simulink library "device_library"  (R2021b)
settings: Solver=VariableStepAuto  StartTime=0.0  StopTime=10.0  RelTol=1e-3
undefined symbols (not defined in the file or in its folder): base
libraries: spsControlledVoltageSourceLib x15, spsThreePhaseVIMeasurementLib x10, spsabctodq0Lib x10, $bdroot x6, spsThreePhaseSeriesRLCBranchLib x5, spsdq0toabcLib x3
settings Model: Creator=lpwoolcock  LastModifiedBy=lukew
settings SolverCC: AlgebraicLoopSolver=TrustRegion
settings DebuggingCC: SFMachineParentedDataDiag=warning

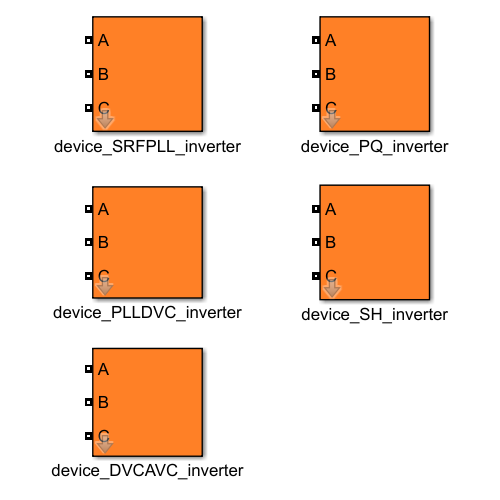
[thumbnail: Simulink's stored preview of the top-level diagram]
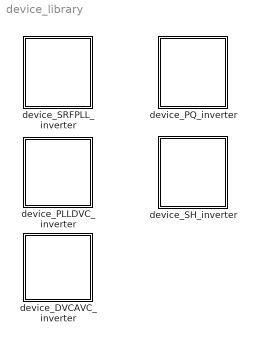
== system device_library ==
  device_DVCAVC_inverter : Subsystem  mask{Rf=0, Lf=0, Cdc=0, K_p_acc=0, K_i_acc=0, K_p_pll=0, K_i_pll=0, K_p_dvc=0, K_i_dvc=0, K_p_avc=0, K_i_avc=0, Psrc=0, Vref=0, K_droop=0}
      mask Display: patch([0 1 1 0], [0 0 1 1], [1 0.5 0.15])
  device_PLLDVC_inverter : Subsystem  mask{Rf=0, Lf=0, K_p_pll=0, K_i_pll=0, K_p_acc=0, K_i_acc=0, K_p_dvc=0, K_i_dvc=0, Psrc=0, Iq=0, Cdc=0}
      mask Display: patch([0 1 1 0], [0 0 1 1], [1 0.5 0.15])
  device_PQ_inverter : Subsystem  mask{Rf=0, Lf=0, S0=0, phi=0, K_p_pll=0, K_i_pll=0, K_p_acc=0, K_i_acc=0, K_p_P=0, K_i_P=0}
      mask Display: patch([0 1 1 0], [0 0 1 1], [1 0.5 0.15])
  device_SH_inverter : Subsystem  mask{Rf=0, Lf=0, P0=0, Q0=0, tau_rms=0, K_p_pll=0, K_i_pll=0, K_p_acc=0, K_i_acc=0}
      mask Display: patch([0 1 1 0], [0 0 1 1], [1 0.5 0.15])
  device_SRFPLL_inverter : Subsystem  mask{Rf=0, Lf=0, Iref=0, phi=0, K_p_pll=0, K_i_pll=0, K_p_acc=0, K_i_acc=0}
      mask prompts: Iref "I0"
      mask Display: patch([0 1 1 0], [0 0 1 1], [1 0.5 0.15])

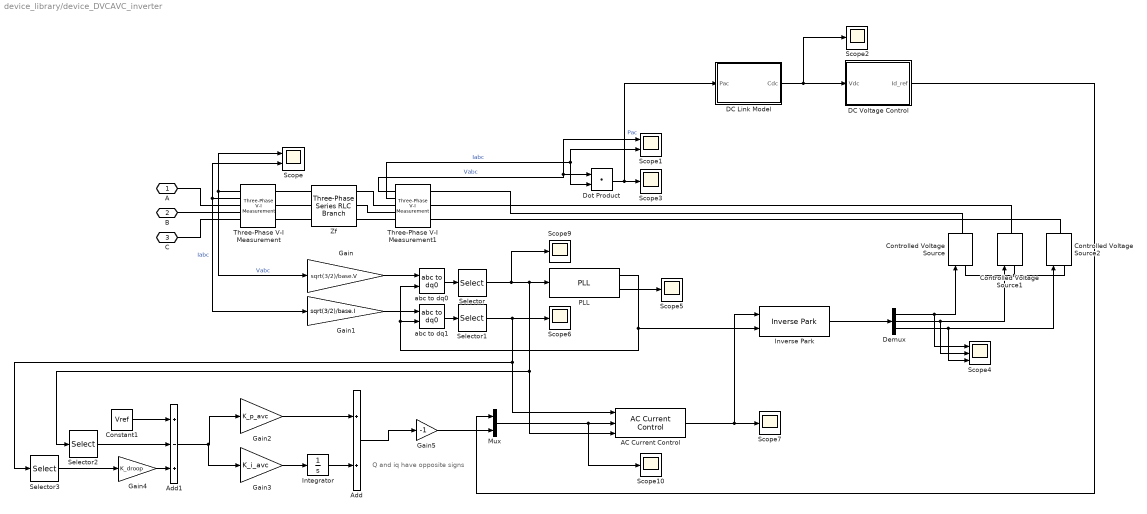
== system device_library/device_DVCAVC_inverter ==
  note: Q and iq have opposite signs
  AC Current Control : $bdroot/device_SRFPLL_inverter/AC Current Control  SystemSampleTime=-1  VariantActivationTime=update diagram  Latency=0  AutoFrameSizeCalculation=off
  Add : Sum
  Add1 : Sum  Inputs=+-+
  Constant1 : Constant  Value=Vref
  Controlled Voltage Source : spsControlledVoltageSourceLib/Controlled Voltage Source  Initialize=on  Source_Type=AC  Amplitude=0  Phase=0  Frequency=0  Measurements=None
  Controlled Voltage Source1 : spsControlledVoltageSourceLib/Controlled Voltage Source  Initialize=on  Source_Type=AC  Amplitude=0  Phase=0  Frequency=0  Measurements=None
  Controlled Voltage Source2 : spsControlledVoltageSourceLib/Controlled Voltage Source  Initialize=on  Source_Type=AC  Amplitude=0  Phase=0  Frequency=0  Measurements=None
  DC Link Model : Subsystem
  DC Voltage Control : Subsystem
  Demux : Demux  Outputs=3
  Dot Product : DotProduct  InputSameDT=on  OutDataTypeStr=Inherit: Inherit via internal rule
  Gain : Gain  Gain=sqrt(3/2)/base.V
  Gain1 : Gain  Gain=sqrt(3/2)/base.I
  Gain2 : Gain  Gain=K_p_avc
  Gain3 : Gain  Gain=K_i_avc
  Gain4 : Gain  Gain=K_droop
  Gain5 : Gain  Gain=-1
  Integrator : Integrator
  Inverse Park : $bdroot/device_SRFPLL_inverter/Inverse Park  SystemSampleTime=-1  VariantActivationTime=update diagram  Latency=0  AutoFrameSizeCalculation=off
  Mux : Mux  Inputs=2
  PLL : $bdroot/device_SRFPLL_inverter/PLL  SystemSampleTime=-1  VariantActivationTime=update diagram  Latency=0  AutoFrameSizeCalculation=off
  Scope : Scope  NumInputPorts=2
  Scope1 : Scope  NumInputPorts=2
  Scope{2..3,5..7,9..10} (7 alike) : Scope
  Scope4 : Scope  NumInputPorts=3
  Selector : Selector  InputPortWidth=3  IndexOptions=Index vector (dialog)  Indices=[1 2]  OutputSizes=1
  Selector1 : Selector  InputPortWidth=3  IndexOptions=Index vector (dialog)  Indices=[1 2]  OutputSizes=1
  Selector2 : Selector  InputPortWidth=2  IndexOptions=Index vector (dialog)  Indices=[1]  OutputSizes=1
  Selector3 : Selector  InputPortWidth=2  IndexOptions=Index vector (dialog)  Indices=[2]  OutputSizes=1
  Three-Phase V-I Measurement : spsThreePhaseVIMeasurementLib/Three-Phase V-I Measurement  VoltageMeasurement=phase-to-ground  SetLabelV=off  LabelV=Vabc  Vpu=off  VpuLL=off  CurrentMeasurement=yes  SetLabelI=off  LabelI=Iabc  Ipu=off  Pbase=100e6  Vbase=500e3  OutputType=Complex  PhasorSimulation=off  PSBequivalent=0
  Three-Phase V-I Measurement1 : spsThreePhaseVIMeasurementLib/Three-Phase V-I Measurement  VoltageMeasurement=phase-to-ground  SetLabelV=off  LabelV=Vabc  Vpu=off  VpuLL=off  CurrentMeasurement=yes  SetLabelI=off  LabelI=Iabc  Ipu=off  Pbase=100e6  Vbase=500e3  OutputType=Complex  PhasorSimulation=off  PSBequivalent=0
  Zf : spsThreePhaseSeriesRLCBranchLib/Three-Phase Series RLC Branch  LConnTagsString=A|B|C  RConnTagsString=A|B|C  BranchType=RL  Resistance=Rf*base.Z  Inductance=Lf*base.L  Capacitance=1e-6  Measurements=None
  abc to dq0 : spsabctodq0Lib/abc to dq0  Alignment=90 degrees behind phase A axis
  abc to dq1 : spsabctodq0Lib/abc to dq0  Alignment=90 degrees behind phase A axis
  "A " : PMIOPort  Side=Left
  B : PMIOPort  Port=2  Side=Left
  C : PMIOPort  Port=3  Side=Left
  wires:
  AC Current Control/1 -> Inverse Park/1, Scope7/1
  Gain1/1 -> abc to dq1/1
  Three-Phase V-I Measurement/1 -> Gain/1, Scope/1  "Vabc"
  DC Voltage Control/1(Id_ref) -> Mux/1
  Add/1 -> Gain5/1
  abc to dq0/1 -> Selector/1
  Gain3/1 -> Integrator/1
  Constant1/1 -> Add1/1
  Dot Product/1 -> Scope3/1, DC Link Model/1(Pac)  "Pac"
  Selector3/1 -> Gain4/1
  Demux/1 -> Controlled Voltage Source/1, Scope4/1
  Selector/1 -> PLL/1, AC Current Control/3, Selector2/1, Scope9/1
  PLL/2 -> Scope5/1
  Three-Phase V-I Measurement/2 -> Gain1/1, Scope/2  "Iabc"
  PLL/1 -> Inverse Park/2, abc to dq0/2, abc to dq1/2
  Demux/3 -> Controlled Voltage Source2/1, Scope4/3
  abc to dq1/1 -> Selector1/1
  Three-Phase V-I Measurement1/2 -> Dot Product/2, Scope1/2  "Iabc"
  Demux/2 -> Controlled Voltage Source1/1, Scope4/2
  Gain5/1 -> Mux/2
  Mux/1 -> AC Current Control/2, Scope10/1
  Three-Phase V-I Measurement1/1 -> Dot Product/1, Scope1/1  "Vabc"
  Gain2/1 -> Add/1
  Gain4/1 -> Add1/3
  Selector2/1 -> Add1/2
  Integrator/1 -> Add/2
  Gain/1 -> abc to dq0/1
  Inverse Park/1 -> Demux/1
  Selector1/1 -> Scope6/1, AC Current Control/1, Selector3/1
  DC Link Model/1(Cdc) -> DC Voltage Control/1(Vdc), Scope2/1
  Add1/1 -> Gain2/1, Gain3/1
  connections:
  Controlled Voltage Source2/LConn1 -- Controlled Voltage Source/LConn1 -- Controlled Voltage Source1/LConn1
  Three-Phase V-I Measurement/LConn3 -- Zf/LConn3
  C/RConn1 -- Three-Phase V-I Measurement/RConn3
  Zf/RConn3 -- Three-Phase V-I Measurement1/RConn3
  Three-Phase V-I Measurement1/LConn2 -- Controlled Voltage Source1/RConn1
  B/RConn1 -- Three-Phase V-I Measurement/RConn2
  Three-Phase V-I Measurement/LConn2 -- Zf/LConn2
  Zf/RConn1 -- Three-Phase V-I Measurement1/RConn1
  Three-Phase V-I Measurement1/LConn3 -- Controlled Voltage Source2/RConn1
  Three-Phase V-I Measurement1/LConn1 -- Controlled Voltage Source/RConn1
  Zf/RConn2 -- Three-Phase V-I Measurement1/RConn2
  "A "/RConn1 -- Three-Phase V-I Measurement/RConn1
  Three-Phase V-I Measurement/LConn1 -- Zf/LConn1

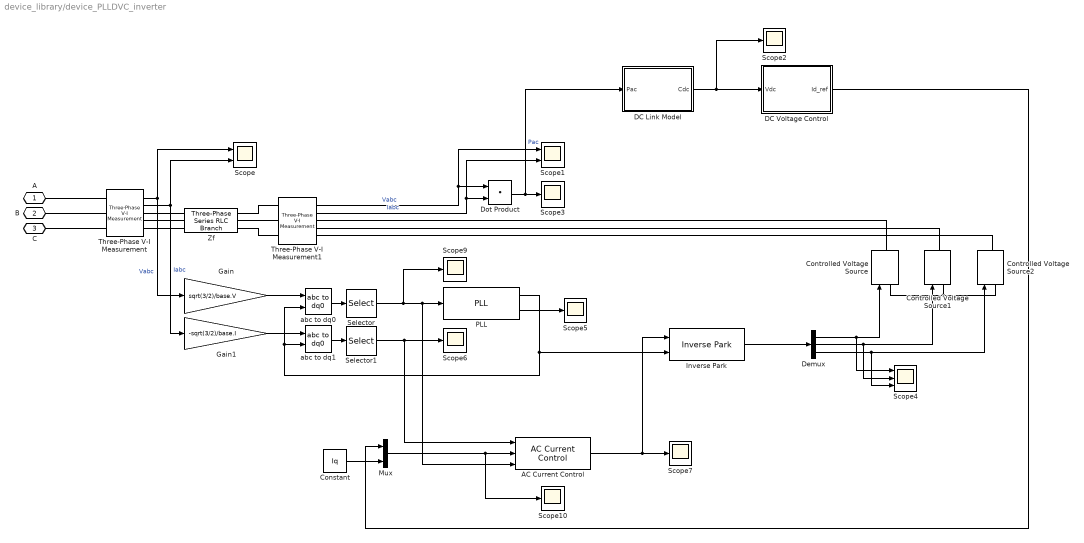
== system device_library/device_PLLDVC_inverter ==
  AC Current Control : $bdroot/device_SRFPLL_inverter/AC Current Control  SystemSampleTime=-1  VariantActivationTime=update diagram  Latency=0  AutoFrameSizeCalculation=off
  Constant : Constant  Value=Iq
  Controlled Voltage Source : spsControlledVoltageSourceLib/Controlled Voltage Source  Initialize=on  Source_Type=AC  Amplitude=0  Phase=0  Frequency=0  Measurements=None
  Controlled Voltage Source1 : spsControlledVoltageSourceLib/Controlled Voltage Source  Initialize=on  Source_Type=AC  Amplitude=0  Phase=0  Frequency=0  Measurements=None
  Controlled Voltage Source2 : spsControlledVoltageSourceLib/Controlled Voltage Source  Initialize=on  Source_Type=AC  Amplitude=0  Phase=0  Frequency=0  Measurements=None
  DC Link Model : Subsystem
  DC Voltage Control : Subsystem
  Demux : Demux  Outputs=3
  Dot Product : DotProduct  InputSameDT=on  OutDataTypeStr=Inherit: Inherit via internal rule
  Gain : Gain  Gain=sqrt(3/2)/base.V
  Gain1 : Gain  Gain=-sqrt(3/2)/base.I
  Inverse Park : $bdroot/device_SRFPLL_inverter/Inverse Park  SystemSampleTime=-1  VariantActivationTime=update diagram  Latency=0  AutoFrameSizeCalculation=off
  Mux : Mux  Inputs=2
  PLL : $bdroot/device_SRFPLL_inverter/PLL  SystemSampleTime=-1  VariantActivationTime=update diagram  Latency=0  AutoFrameSizeCalculation=off
  Scope : Scope  NumInputPorts=2
  Scope1 : Scope  NumInputPorts=2
  Scope{2..3,5..7,9..10} (7 alike) : Scope
  Scope4 : Scope  NumInputPorts=3
  Selector : Selector  InputPortWidth=3  IndexOptions=Index vector (dialog)  Indices=[1 2]  OutputSizes=1
  Selector1 : Selector  InputPortWidth=3  IndexOptions=Index vector (dialog)  Indices=[1 2]  OutputSizes=1
  Three-Phase V-I Measurement : spsThreePhaseVIMeasurementLib/Three-Phase V-I Measurement  VoltageMeasurement=phase-to-ground  SetLabelV=off  LabelV=Vabc  Vpu=off  VpuLL=off  CurrentMeasurement=yes  SetLabelI=off  LabelI=Iabc  Ipu=off  Pbase=100e6  Vbase=500e3  OutputType=Complex  PhasorSimulation=off  PSBequivalent=0
  Three-Phase V-I Measurement1 : spsThreePhaseVIMeasurementLib/Three-Phase V-I Measurement  VoltageMeasurement=phase-to-ground  SetLabelV=off  LabelV=Vabc  Vpu=off  VpuLL=off  CurrentMeasurement=yes  SetLabelI=off  LabelI=Iabc  Ipu=off  Pbase=100e6  Vbase=500e3  OutputType=Complex  PhasorSimulation=off  PSBequivalent=0
  Zf : spsThreePhaseSeriesRLCBranchLib/Three-Phase Series RLC Branch  LConnTagsString=A|B|C  RConnTagsString=A|B|C  BranchType=RL  Resistance=Rf*base.Z  Inductance=Lf*base.L  Capacitance=1e-6  Measurements=None
  abc to dq0 : spsabctodq0Lib/abc to dq0  Alignment=90 degrees behind phase A axis
  abc to dq1 : spsabctodq0Lib/abc to dq0  Alignment=90 degrees behind phase A axis
  "A " : PMIOPort  Side=Left
  B : PMIOPort  Port=2  Side=Left
  C : PMIOPort  Port=3  Side=Left
  wires:
  Constant/1 -> Mux/2
  Selector1/1 -> AC Current Control/1, Scope6/1
  AC Current Control/1 -> Scope7/1, Inverse Park/1
  Mux/1 -> Scope10/1, AC Current Control/2
  Inverse Park/1 -> Demux/1
  Demux/3 -> Scope4/3, Controlled Voltage Source2/1
  Three-Phase V-I Measurement/1 -> Gain/1, Scope/1  "Vabc"
  PLL/1 -> abc to dq1/2, abc to dq0/2, Inverse Park/2
  PLL/2 -> Scope5/1
  Dot Product/1 -> DC Link Model/1(Pac), Scope3/1  "Pac"
  Demux/1 -> Scope4/1, Controlled Voltage Source/1
  Three-Phase V-I Measurement1/1 -> Scope1/1, Dot Product/1  "Vabc"
  DC Link Model/1(Cdc) -> Scope2/1, DC Voltage Control/1(Vdc)
  Three-Phase V-I Measurement/2 -> Scope/2, Gain1/1  "Iabc"
  DC Voltage Control/1(Id_ref) -> Mux/1
  Demux/2 -> Scope4/2, Controlled Voltage Source1/1
  Three-Phase V-I Measurement1/2 -> Dot Product/2, Scope1/2  "Iabc"
  Gain1/1 -> abc to dq1/1
  Gain/1 -> abc to dq0/1
  Selector/1 -> Scope9/1, AC Current Control/3, PLL/1
  abc to dq0/1 -> Selector/1
  abc to dq1/1 -> Selector1/1
  connections:
  Controlled Voltage Source2/LConn1 -- Controlled Voltage Source1/LConn1 -- Controlled Voltage Source/LConn1
  Three-Phase V-I Measurement1/LConn1 -- Zf/RConn1
  B/RConn1 -- Three-Phase V-I Measurement/LConn2
  Three-Phase V-I Measurement/RConn2 -- Zf/LConn2
  Three-Phase V-I Measurement1/RConn2 -- Controlled Voltage Source1/RConn1
  "A "/RConn1 -- Three-Phase V-I Measurement/LConn1
  C/RConn1 -- Three-Phase V-I Measurement/LConn3
  Three-Phase V-I Measurement1/RConn1 -- Controlled Voltage Source/RConn1
  Three-Phase V-I Measurement1/RConn3 -- Controlled Voltage Source2/RConn1
  Zf/RConn3 -- Three-Phase V-I Measurement1/LConn3
  Zf/RConn2 -- Three-Phase V-I Measurement1/LConn2
  Zf/LConn1 -- Three-Phase V-I Measurement/RConn1
  Three-Phase V-I Measurement/RConn3 -- Zf/LConn3

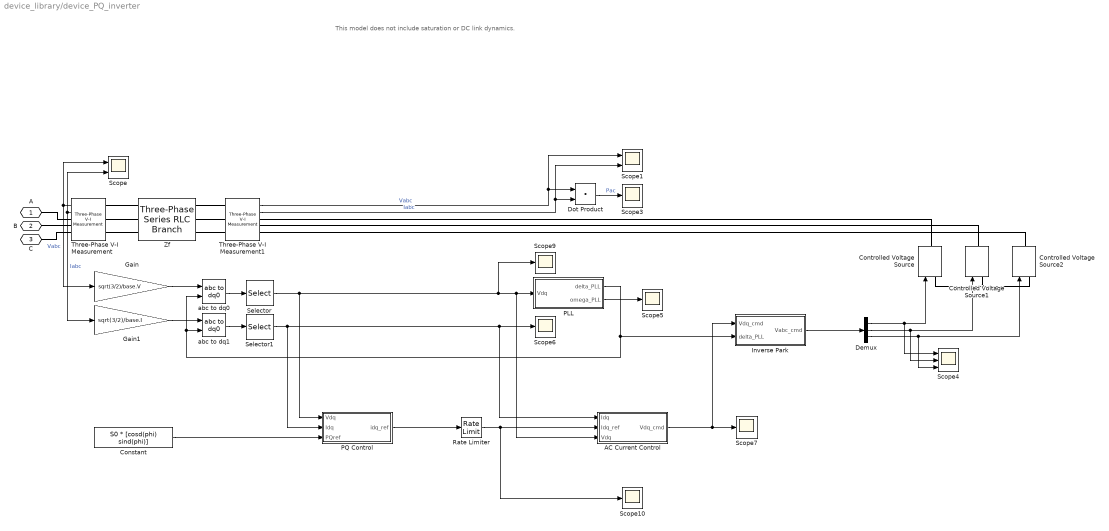
== system device_library/device_PQ_inverter ==
  note: This model does not include saturation or DC link dynamics.
  AC Current Control : Subsystem
  Constant : Constant  Value=S0 * [cosd(phi) sind(phi)]
  Controlled Voltage Source : spsControlledVoltageSourceLib/Controlled Voltage Source  Initialize=on  Source_Type=AC  Amplitude=0  Phase=0  Frequency=0  Measurements=None
  Controlled Voltage Source1 : spsControlledVoltageSourceLib/Controlled Voltage Source  Initialize=on  Source_Type=AC  Amplitude=0  Phase=0  Frequency=0  Measurements=None
  Controlled Voltage Source2 : spsControlledVoltageSourceLib/Controlled Voltage Source  Initialize=on  Source_Type=AC  Amplitude=0  Phase=0  Frequency=0  Measurements=None
  Demux : Demux  Outputs=3
  Dot Product : DotProduct  InputSameDT=on  OutDataTypeStr=Inherit: Inherit via internal rule
  Gain : Gain  Gain=sqrt(3/2)/base.V
  Gain1 : Gain  Gain=sqrt(3/2)/base.I
  Inverse Park : Subsystem
  PLL : Subsystem
  PQ Control : Subsystem
  Rate Limiter : RateLimiter  RisingSlewLimit=1000  FallingSlewLimit=-1000  SampleTimeMode=inherited
  Scope : Scope  NumInputPorts=2
  Scope1 : Scope  NumInputPorts=2
  Scope{3,5..7,9..10} (6 alike) : Scope
  Scope4 : Scope  NumInputPorts=3
  Selector : Selector  InputPortWidth=3  IndexOptions=Index vector (dialog)  Indices=[1 2]  OutputSizes=1
  Selector1 : Selector  InputPortWidth=3  IndexOptions=Index vector (dialog)  Indices=[1 2]  OutputSizes=1
  Three-Phase V-I Measurement : spsThreePhaseVIMeasurementLib/Three-Phase V-I Measurement  VoltageMeasurement=phase-to-ground  SetLabelV=off  LabelV=Vabc  Vpu=off  VpuLL=off  CurrentMeasurement=yes  SetLabelI=off  LabelI=Iabc  Ipu=off  Pbase=100e6  Vbase=500e3  OutputType=Complex  PhasorSimulation=off  PSBequivalent=0
  Three-Phase V-I Measurement1 : spsThreePhaseVIMeasurementLib/Three-Phase V-I Measurement  VoltageMeasurement=phase-to-ground  SetLabelV=off  LabelV=Vabc  Vpu=off  VpuLL=off  CurrentMeasurement=yes  SetLabelI=off  LabelI=Iabc  Ipu=off  Pbase=100e6  Vbase=500e3  OutputType=Complex  PhasorSimulation=off  PSBequivalent=0
  Zf : spsThreePhaseSeriesRLCBranchLib/Three-Phase Series RLC Branch  LConnTagsString=A|B|C  RConnTagsString=A|B|C  BranchType=RL  Resistance=Rf*base.Z  Inductance=Lf*base.L  Capacitance=1e-6  Measurements=None
  abc to dq0 : spsabctodq0Lib/abc to dq0  Alignment=90 degrees behind phase A axis
  abc to dq1 : spsabctodq0Lib/abc to dq0  Alignment=90 degrees behind phase A axis
  A : PMIOPort  Side=Left
  B : PMIOPort  Port=2  Side=Left
  C : PMIOPort  Port=3  Side=Left
  wires:
  Rate Limiter/1 -> AC Current Control/2(Idq_ref), Scope10/1
  Inverse Park/1(Vabc_cmd) -> Demux/1
  abc to dq1/1 -> Selector1/1
  PLL/2(omega_PLL) -> Scope5/1
  abc to dq0/1 -> Selector/1
  Three-Phase V-I Measurement1/1 -> Dot Product/1, Scope1/1  "Vabc"
  Gain/1 -> abc to dq0/1
  Demux/3 -> Controlled Voltage Source2/1, Scope4/3
  Three-Phase V-I Measurement1/2 -> Scope1/2, Dot Product/2  "Iabc"
  AC Current Control/1(Vdq_cmd) -> Inverse Park/1(Vdq_cmd), Scope7/1
  Selector1/1 -> PQ Control/2(Idq), Scope6/1, AC Current Control/1(Idq)
  Dot Product/1 -> Scope3/1  "Pac"
  Demux/1 -> Controlled Voltage Source/1, Scope4/1
  Three-Phase V-I Measurement/1 -> Scope/1, Gain/1  "Vabc"
  Demux/2 -> Controlled Voltage Source1/1, Scope4/2
  Gain1/1 -> abc to dq1/1
  Three-Phase V-I Measurement/2 -> Scope/2, Gain1/1  "Iabc"
  PLL/1(delta_PLL) -> Inverse Park/2(delta_PLL), abc to dq0/2, abc to dq1/2
  Selector/1 -> PQ Control/1(Vdq), PLL/1(Vdq), AC Current Control/3(Vdq), Scope9/1
  Constant/1 -> PQ Control/3(PQref)
  PQ Control/1(idq_ref) -> Rate Limiter/1
  connections:
  Three-Phase V-I Measurement1/LConn1 -- Zf/RConn1
  Three-Phase V-I Measurement1/RConn2 -- Controlled Voltage Source1/RConn1
  Controlled Voltage Source2/LConn1 -- Controlled Voltage Source1/LConn1 -- Controlled Voltage Source/LConn1
  Three-Phase V-I Measurement1/RConn3 -- Controlled Voltage Source2/RConn1
  Zf/RConn3 -- Three-Phase V-I Measurement1/LConn3
  Zf/RConn2 -- Three-Phase V-I Measurement1/LConn2
  Three-Phase V-I Measurement1/RConn1 -- Controlled Voltage Source/RConn1
  A/RConn1 -- Three-Phase V-I Measurement/RConn1
  B/RConn1 -- Three-Phase V-I Measurement/RConn2
  C/RConn1 -- Three-Phase V-I Measurement/RConn3
  Three-Phase V-I Measurement/LConn1 -- Zf/LConn1
  Three-Phase V-I Measurement/LConn2 -- Zf/LConn2
  Three-Phase V-I Measurement/LConn3 -- Zf/LConn3

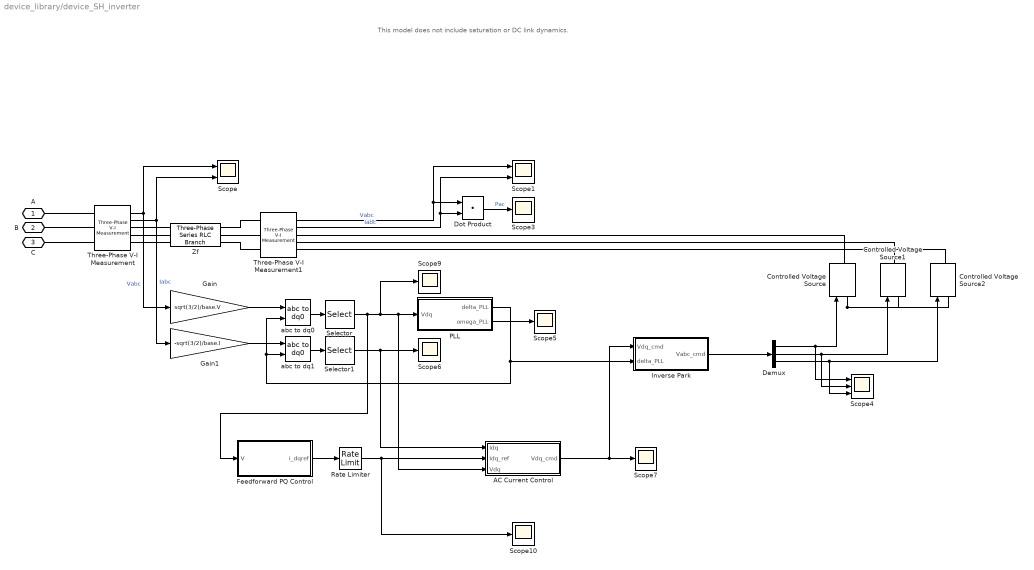
== system device_library/device_SH_inverter ==
  note: This model does not include saturation or DC link dynamics.
  AC Current Control : Subsystem
  Controlled Voltage Source : spsControlledVoltageSourceLib/Controlled Voltage Source  Initialize=on  Source_Type=AC  Amplitude=0  Phase=0  Frequency=0  Measurements=None
  Controlled Voltage Source1 : spsControlledVoltageSourceLib/Controlled Voltage Source  Initialize=on  Source_Type=AC  Amplitude=0  Phase=0  Frequency=0  Measurements=None
  Controlled Voltage Source2 : spsControlledVoltageSourceLib/Controlled Voltage Source  Initialize=on  Source_Type=AC  Amplitude=0  Phase=0  Frequency=0  Measurements=None
  Demux : Demux  Outputs=3
  Dot Product : DotProduct  InputSameDT=on  OutDataTypeStr=Inherit: Inherit via internal rule
  Feedforward PQ Control : Subsystem
  Gain : Gain  Gain=sqrt(3/2)/base.V
  Gain1 : Gain  Gain=-sqrt(3/2)/base.I
  Inverse Park : Subsystem
  PLL : Subsystem
  Rate Limiter : RateLimiter  RisingSlewLimit=1000  FallingSlewLimit=-1000  SampleTimeMode=inherited
  Scope : Scope  NumInputPorts=2
  Scope1 : Scope  NumInputPorts=2
  Scope{3,5..7,9..10} (6 alike) : Scope
  Scope4 : Scope  NumInputPorts=3
  Selector : Selector  InputPortWidth=3  IndexOptions=Index vector (dialog)  Indices=[1 2]  OutputSizes=1
  Selector1 : Selector  InputPortWidth=3  IndexOptions=Index vector (dialog)  Indices=[1 2]  OutputSizes=1
  Three-Phase V-I Measurement : spsThreePhaseVIMeasurementLib/Three-Phase V-I Measurement  VoltageMeasurement=phase-to-ground  SetLabelV=off  LabelV=Vabc  Vpu=off  VpuLL=off  CurrentMeasurement=yes  SetLabelI=off  LabelI=Iabc  Ipu=off  Pbase=100e6  Vbase=500e3  OutputType=Complex  PhasorSimulation=off  PSBequivalent=0
  Three-Phase V-I Measurement1 : spsThreePhaseVIMeasurementLib/Three-Phase V-I Measurement  VoltageMeasurement=phase-to-ground  SetLabelV=off  LabelV=Vabc  Vpu=off  VpuLL=off  CurrentMeasurement=yes  SetLabelI=off  LabelI=Iabc  Ipu=off  Pbase=100e6  Vbase=500e3  OutputType=Complex  PhasorSimulation=off  PSBequivalent=0
  Zf : spsThreePhaseSeriesRLCBranchLib/Three-Phase Series RLC Branch  LConnTagsString=A|B|C  RConnTagsString=A|B|C  BranchType=RL  Resistance=Rf*base.Z  Inductance=Lf*base.L  Capacitance=1e-6  Measurements=None
  abc to dq0 : spsabctodq0Lib/abc to dq0  Alignment=90 degrees behind phase A axis
  abc to dq1 : spsabctodq0Lib/abc to dq0  Alignment=90 degrees behind phase A axis
  A : PMIOPort  Side=Left
  B : PMIOPort  Port=2  Side=Left
  C : PMIOPort  Port=3  Side=Left
  wires:
  Selector/1 -> Feedforward PQ Control/1(V), Scope9/1, AC Current Control/3(Vdq), PLL/1(Vdq)
  PLL/1(delta_PLL) -> abc to dq1/2, abc to dq0/2, Inverse Park/2(delta_PLL)
  Three-Phase V-I Measurement/2 -> Scope/2, Gain1/1  "Iabc"
  Gain1/1 -> abc to dq1/1
  Demux/2 -> Scope4/2, Controlled Voltage Source1/1
  Three-Phase V-I Measurement/1 -> Gain/1, Scope/1  "Vabc"
  Demux/1 -> Scope4/1, Controlled Voltage Source/1
  Dot Product/1 -> Scope3/1  "Pac"
  Selector1/1 -> AC Current Control/1(Idq), Scope6/1
  AC Current Control/1(Vdq_cmd) -> Scope7/1, Inverse Park/1(Vdq_cmd)
  Three-Phase V-I Measurement1/2 -> Dot Product/2, Scope1/2  "Iabc"
  Demux/3 -> Scope4/3, Controlled Voltage Source2/1
  Gain/1 -> abc to dq0/1
  Three-Phase V-I Measurement1/1 -> Scope1/1, Dot Product/1  "Vabc"
  abc to dq0/1 -> Selector/1
  PLL/2(omega_PLL) -> Scope5/1
  abc to dq1/1 -> Selector1/1
  Inverse Park/1(Vabc_cmd) -> Demux/1
  Rate Limiter/1 -> Scope10/1, AC Current Control/2(Idq_ref)
  Feedforward PQ Control/1(i_dqref) -> Rate Limiter/1
  connections:
  Three-Phase V-I Measurement1/RConn1 -- Controlled Voltage Source/RConn1
  A/RConn1 -- Three-Phase V-I Measurement/LConn1
  Zf/RConn2 -- Three-Phase V-I Measurement1/LConn2
  Three-Phase V-I Measurement/RConn2 -- Zf/LConn2
  B/RConn1 -- Three-Phase V-I Measurement/LConn2
  Zf/RConn3 -- Three-Phase V-I Measurement1/LConn3
  Three-Phase V-I Measurement1/RConn3 -- Controlled Voltage Source2/RConn1
  C/RConn1 -- Three-Phase V-I Measurement/LConn3
  Controlled Voltage Source/LConn1 -- Controlled Voltage Source1/LConn1 -- Controlled Voltage Source2/LConn1
  Three-Phase V-I Measurement1/RConn2 -- Controlled Voltage Source1/RConn1
  Zf/LConn1 -- Three-Phase V-I Measurement/RConn1
  Three-Phase V-I Measurement1/LConn1 -- Zf/RConn1
  Three-Phase V-I Measurement/RConn3 -- Zf/LConn3

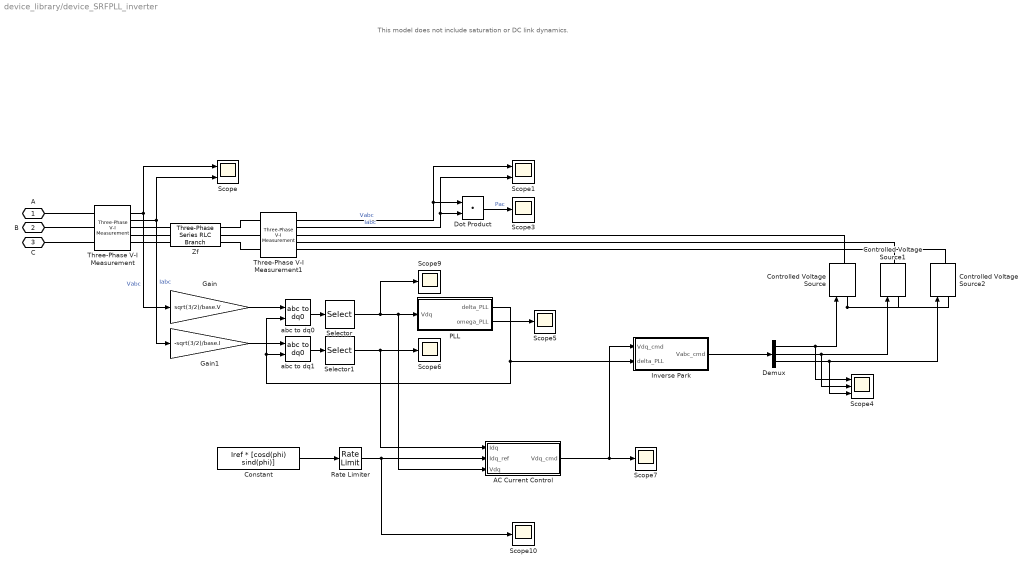
== system device_library/device_SRFPLL_inverter ==
  note: This model does not include saturation or DC link dynamics.
  AC Current Control : Subsystem
  Constant : Constant  Value=Iref * [cosd(phi) sind(phi)]
  Controlled Voltage Source : spsControlledVoltageSourceLib/Controlled Voltage Source  Initialize=on  Source_Type=AC  Amplitude=0  Phase=0  Frequency=0  Measurements=None
  Controlled Voltage Source1 : spsControlledVoltageSourceLib/Controlled Voltage Source  Initialize=on  Source_Type=AC  Amplitude=0  Phase=0  Frequency=0  Measurements=None
  Controlled Voltage Source2 : spsControlledVoltageSourceLib/Controlled Voltage Source  Initialize=on  Source_Type=AC  Amplitude=0  Phase=0  Frequency=0  Measurements=None
  Demux : Demux  Outputs=3
  Dot Product : DotProduct  InputSameDT=on  OutDataTypeStr=Inherit: Inherit via internal rule
  Gain : Gain  Gain=sqrt(3/2)/base.V
  Gain1 : Gain  Gain=-sqrt(3/2)/base.I
  Inverse Park : Subsystem
  PLL : Subsystem
  Rate Limiter : RateLimiter  RisingSlewLimit=1000  FallingSlewLimit=-1000  SampleTimeMode=inherited
  Scope : Scope  NumInputPorts=2
  Scope1 : Scope  NumInputPorts=2
  Scope{3,5..7,9..10} (6 alike) : Scope
  Scope4 : Scope  NumInputPorts=3
  Selector : Selector  InputPortWidth=3  IndexOptions=Index vector (dialog)  Indices=[1 2]  OutputSizes=1
  Selector1 : Selector  InputPortWidth=3  IndexOptions=Index vector (dialog)  Indices=[1 2]  OutputSizes=1
  Three-Phase V-I Measurement : spsThreePhaseVIMeasurementLib/Three-Phase V-I Measurement  VoltageMeasurement=phase-to-ground  SetLabelV=off  LabelV=Vabc  Vpu=off  VpuLL=off  CurrentMeasurement=yes  SetLabelI=off  LabelI=Iabc  Ipu=off  Pbase=100e6  Vbase=500e3  OutputType=Complex  PhasorSimulation=off  PSBequivalent=0
  Three-Phase V-I Measurement1 : spsThreePhaseVIMeasurementLib/Three-Phase V-I Measurement  VoltageMeasurement=phase-to-ground  SetLabelV=off  LabelV=Vabc  Vpu=off  VpuLL=off  CurrentMeasurement=yes  SetLabelI=off  LabelI=Iabc  Ipu=off  Pbase=100e6  Vbase=500e3  OutputType=Complex  PhasorSimulation=off  PSBequivalent=0
  Zf : spsThreePhaseSeriesRLCBranchLib/Three-Phase Series RLC Branch  LConnTagsString=A|B|C  RConnTagsString=A|B|C  BranchType=RL  Resistance=Rf*base.Z  Inductance=Lf*base.L  Capacitance=1e-6  Measurements=None
  abc to dq0 : spsabctodq0Lib/abc to dq0  Alignment=90 degrees behind phase A axis
  abc to dq1 : spsabctodq0Lib/abc to dq0  Alignment=90 degrees behind phase A axis
  A : PMIOPort  Side=Left
  B : PMIOPort  Port=2  Side=Left
  C : PMIOPort  Port=3  Side=Left
  wires:
  Selector/1 -> Scope9/1, AC Current Control/3(Vdq), PLL/1(Vdq)
  PLL/1(delta_PLL) -> abc to dq1/2, abc to dq0/2, Inverse Park/2(delta_PLL)
  Three-Phase V-I Measurement/2 -> Scope/2, Gain1/1  "Iabc"
  Gain1/1 -> abc to dq1/1
  Demux/2 -> Scope4/2, Controlled Voltage Source1/1
  Three-Phase V-I Measurement/1 -> Gain/1, Scope/1  "Vabc"
  Demux/1 -> Scope4/1, Controlled Voltage Source/1
  Dot Product/1 -> Scope3/1  "Pac"
  Selector1/1 -> AC Current Control/1(Idq), Scope6/1
  AC Current Control/1(Vdq_cmd) -> Scope7/1, Inverse Park/1(Vdq_cmd)
  Three-Phase V-I Measurement1/2 -> Dot Product/2, Scope1/2  "Iabc"
  Demux/3 -> Scope4/3, Controlled Voltage Source2/1
  Gain/1 -> abc to dq0/1
  Three-Phase V-I Measurement1/1 -> Scope1/1, Dot Product/1  "Vabc"
  abc to dq0/1 -> Selector/1
  PLL/2(omega_PLL) -> Scope5/1
  abc to dq1/1 -> Selector1/1
  Inverse Park/1(Vabc_cmd) -> Demux/1
  Constant/1 -> Rate Limiter/1
  Rate Limiter/1 -> Scope10/1, AC Current Control/2(Idq_ref)
  connections:
  Three-Phase V-I Measurement1/RConn1 -- Controlled Voltage Source/RConn1
  A/RConn1 -- Three-Phase V-I Measurement/LConn1
  Zf/RConn2 -- Three-Phase V-I Measurement1/LConn2
  Three-Phase V-I Measurement/RConn2 -- Zf/LConn2
  B/RConn1 -- Three-Phase V-I Measurement/LConn2
  Zf/RConn3 -- Three-Phase V-I Measurement1/LConn3
  Three-Phase V-I Measurement1/RConn3 -- Controlled Voltage Source2/RConn1
  C/RConn1 -- Three-Phase V-I Measurement/LConn3
  Controlled Voltage Source/LConn1 -- Controlled Voltage Source1/LConn1 -- Controlled Voltage Source2/LConn1
  Three-Phase V-I Measurement1/RConn2 -- Controlled Voltage Source1/RConn1
  Zf/LConn1 -- Three-Phase V-I Measurement/RConn1
  Three-Phase V-I Measurement1/LConn1 -- Zf/RConn1
  Three-Phase V-I Measurement/RConn3 -- Zf/LConn3

== system device_library/device_DVCAVC_inverter/DC Link Model ==
  Pac : Inport
  Add : Sum  Inputs=-+
  Constant1 : Constant  Value=Psrc
  Divide : Product  Inputs=*/
  Gain2 : Gain  Gain=base.omega/Cdc
  Gain3 : Gain  Gain=1/base.S
  Integrator : Integrator  InitialCondition=1
  Scope2 : Scope
  Scope8 : Scope
  Cdc : Outport
  wires:
  Gain3/1 -> Add/1
  Gain2/1 -> Integrator/1
  Divide/1 -> Gain2/1
  Constant1/1 -> Add/2
  Add/1 -> Divide/1, Scope8/1
  Integrator/1 -> Divide/2, Scope2/1, Cdc/1
  Pac/1 -> Gain3/1

== system device_library/device_DVCAVC_inverter/DC Voltage Control ==
  Vdc : Inport
  Add : Sum  Inputs=-+
  Add1 : Sum
  Constant1 : Constant
  Gain2 : Gain  Gain=K_p_dvc
  Gain3 : Gain  Gain=K_i_dvc
  Integrator : Integrator  InitialCondition=Psrc
  Id_ref : Outport
  wires:
  Constant1/1 -> Add/1
  Add1/1 -> Id_ref/1
  Integrator/1 -> Add1/2
  Vdc/1 -> Add/2
  Add/1 -> Gain3/1, Gain2/1
  Gain3/1 -> Integrator/1
  Gain2/1 -> Add1/1

== system device_library/device_PLLDVC_inverter/DC Link Model ==
  Pac : Inport
  Add : Sum  Inputs=-+
  Constant1 : Constant  Value=Psrc
  Divide : Product  Inputs=*/
  Gain2 : Gain  Gain=base.omega/Cdc
  Gain3 : Gain  Gain=-1/base.S
  Integrator : Integrator  InitialCondition=1
  Scope2 : Scope
  Scope8 : Scope
  Cdc : Outport
  wires:
  Pac/1 -> Gain3/1
  Integrator/1 -> Cdc/1, Scope2/1, Divide/2
  Add/1 -> Scope8/1, Divide/1
  Constant1/1 -> Add/2
  Divide/1 -> Gain2/1
  Gain2/1 -> Integrator/1
  Gain3/1 -> Add/1

== system device_library/device_PLLDVC_inverter/DC Voltage Control ==
  Vdc : Inport
  Add : Sum  Inputs=-+
  Add1 : Sum
  Constant1 : Constant
  Gain2 : Gain  Gain=K_p_dvc
  Gain3 : Gain  Gain=K_i_dvc
  Integrator : Integrator  InitialCondition=Psrc
  Id_ref : Outport
  wires:
  Gain2/1 -> Add1/1
  Gain3/1 -> Integrator/1
  Add/1 -> Gain2/1, Gain3/1
  Vdc/1 -> Add/2
  Integrator/1 -> Add1/2
  Add1/1 -> Id_ref/1
  Constant1/1 -> Add/1

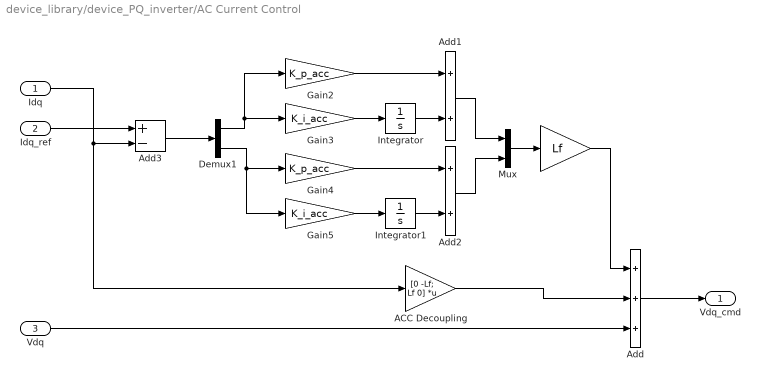
== system device_library/device_PQ_inverter/AC Current Control ==
  Idq : Inport
  Idq_ref : Inport  Port=2
  Vdq : Inport  Port=3
  "  " : Gain  Gain=Lf
  ACC Decoupling : Gain  Gain=[0 -Lf; Lf 0]  Multiplication=Matrix(K*u) (u vector)
  Add : Sum  Inputs=3
  Add1 : Sum
  Add2 : Sum
  Add3 : Sum  Inputs=+-
  Demux1 : Demux  Outputs=2
  Gain2 : Gain  Gain=K_p_acc
  Gain3 : Gain  Gain=K_i_acc
  Gain4 : Gain  Gain=K_p_acc
  Gain5 : Gain  Gain=K_i_acc
  Integrator : Integrator
  Integrator1 : Integrator
  Mux : Mux  Inputs=2
  Vdq_cmd : Outport
  wires:
  Vdq/1 -> Add/3
  ACC Decoupling/1 -> Add/2
  Idq_ref/1 -> Add3/1
  Idq/1 -> Add3/2, ACC Decoupling/1
  Add/1 -> Vdq_cmd/1
  Demux1/1 -> Gain2/1, Gain3/1
  Integrator1/1 -> Add2/2
  Integrator/1 -> Add1/2
  Gain2/1 -> Add1/1
  Add1/1 -> Mux/1
  Gain3/1 -> Integrator/1
  Gain5/1 -> Integrator1/1
  Add2/1 -> Mux/2
  Gain4/1 -> Add2/1
  Add3/1 -> Demux1/1
  Demux1/2 -> Gain5/1, Gain4/1
  Mux/1 -> "  "/1
  "  "/1 -> Add/1

== system device_library/device_PQ_inverter/Inverse Park ==
  Vdq_cmd : Inport
  delta_PLL : Inport  Port=2
  Constant : Constant  Value=0
  Gain : Gain  Gain=base.V*sqrt(2/3)
  Mux : Mux  Inputs=2
  dq0 to abc : spsdq0toabcLib/dq0 to abc  Alignment=90 degrees behind phase A axis
  Vabc_cmd : Outport
  wires:
  Vdq_cmd/1 -> Mux/1
  Constant/1 -> Mux/2
  Gain/1 -> Vabc_cmd/1
  dq0 to abc/1 -> Gain/1
  delta_PLL/1 -> dq0 to abc/2
  Mux/1 -> dq0 to abc/1

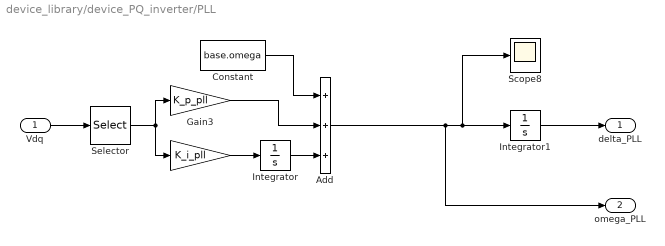
== system device_library/device_PQ_inverter/PLL ==
  Vdq : Inport
  " " : Gain  Gain=K_i_pll
  Add : Sum  Inputs=+++
  Constant : Constant  Value=base.omega
  Gain3 : Gain  Gain=K_p_pll
  Integrator : Integrator
  Integrator1 : Integrator
  Scope8 : Scope
  Selector : Selector  InputPortWidth=2  IndexOptions=Index vector (dialog)  Indices=[2]  OutputSizes=1
  delta_PLL : Outport
  omega_PLL : Outport  Port=2
  wires:
  Constant/1 -> Add/1
  Gain3/1 -> Add/2
  Integrator1/1 -> delta_PLL/1
  Vdq/1 -> Selector/1
  " "/1 -> Integrator/1
  Selector/1 -> " "/1, Gain3/1
  Integrator/1 -> Add/3
  Add/1 -> Integrator1/1, Scope8/1, omega_PLL/1

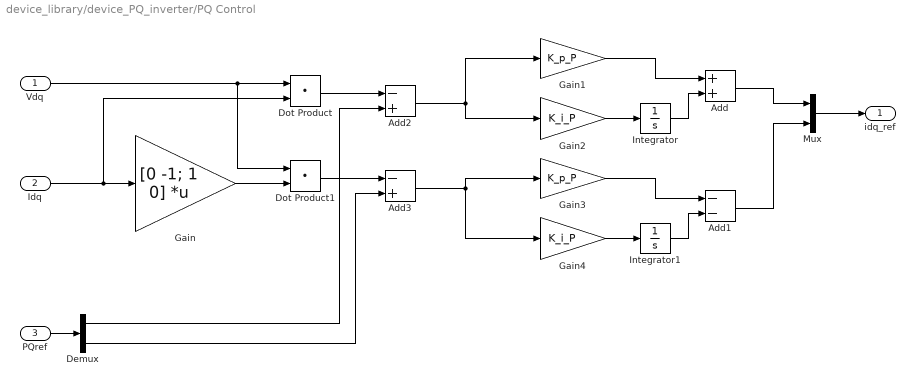
== system device_library/device_PQ_inverter/PQ Control ==
  Vdq : Inport
  Idq : Inport  Port=2
  PQref : Inport  Port=3
  Add : Sum
  Add1 : Sum  Inputs=--
  Add2 : Sum  Inputs=-+
  Add3 : Sum  Inputs=-+
  Demux : Demux  Outputs=2
  Dot Product : DotProduct  InputSameDT=on  OutDataTypeStr=Inherit: Inherit via internal rule
  Dot Product1 : DotProduct  InputSameDT=on  OutDataTypeStr=Inherit: Inherit via internal rule
  Gain : Gain  Gain=[0 -1; 1 0]  Multiplication=Matrix(K*u) (u vector)
  Gain1 : Gain  Gain=K_p_P
  Gain2 : Gain  Gain=K_i_P
  Gain3 : Gain  Gain=K_p_P
  Gain4 : Gain  Gain=K_i_P
  Integrator : Integrator
  Integrator1 : Integrator
  Mux : Mux  Inputs=2
  idq_ref : Outport
  wires:
  Vdq/1 -> Dot Product1/1, Dot Product/1
  Idq/1 -> Gain/1, Dot Product/2
  Gain/1 -> Dot Product1/2
  Gain2/1 -> Integrator/1
  Gain1/1 -> Add/1
  Integrator/1 -> Add/2
  Add/1 -> Mux/1
  Gain3/1 -> Add1/1
  Integrator1/1 -> Add1/2
  Gain4/1 -> Integrator1/1
  Add1/1 -> Mux/2
  Mux/1 -> idq_ref/1
  PQref/1 -> Demux/1
  Dot Product/1 -> Add2/1
  Add2/1 -> Gain2/1, Gain1/1
  Demux/1 -> Add2/2
  Demux/2 -> Add3/2
  Add3/1 -> Gain4/1, Gain3/1
  Dot Product1/1 -> Add3/1

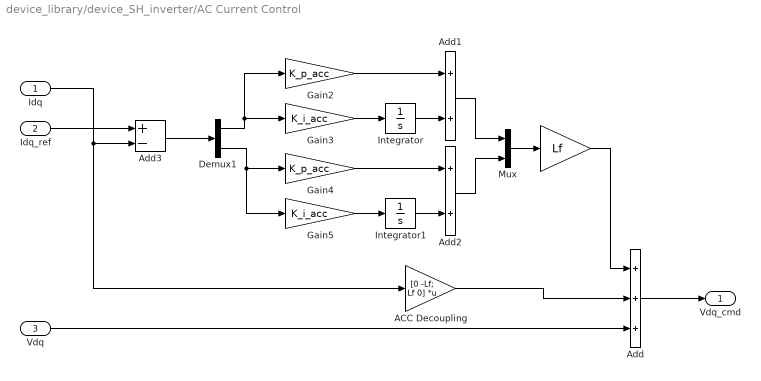
== system device_library/device_SH_inverter/AC Current Control ==
  Idq : Inport
  Idq_ref : Inport  Port=2
  Vdq : Inport  Port=3
  "  " : Gain  Gain=Lf
  ACC Decoupling : Gain  Gain=[0 -Lf; Lf 0]  Multiplication=Matrix(K*u) (u vector)
  Add : Sum  Inputs=3
  Add1 : Sum
  Add2 : Sum
  Add3 : Sum  Inputs=+-
  Demux1 : Demux  Outputs=2
  Gain2 : Gain  Gain=K_p_acc
  Gain3 : Gain  Gain=K_i_acc
  Gain4 : Gain  Gain=K_p_acc
  Gain5 : Gain  Gain=K_i_acc
  Integrator : Integrator
  Integrator1 : Integrator
  Mux : Mux  Inputs=2
  Vdq_cmd : Outport
  wires:
  "  "/1 -> Add/1
  Mux/1 -> "  "/1
  Demux1/2 -> Gain4/1, Gain5/1
  Add3/1 -> Demux1/1
  Gain4/1 -> Add2/1
  Add2/1 -> Mux/2
  Gain5/1 -> Integrator1/1
  Gain3/1 -> Integrator/1
  Add1/1 -> Mux/1
  Gain2/1 -> Add1/1
  Integrator/1 -> Add1/2
  Integrator1/1 -> Add2/2
  Demux1/1 -> Gain3/1, Gain2/1
  Add/1 -> Vdq_cmd/1
  Idq/1 -> ACC Decoupling/1, Add3/2
  Idq_ref/1 -> Add3/1
  ACC Decoupling/1 -> Add/2
  Vdq/1 -> Add/3

== system device_library/device_SH_inverter/Feedforward PQ Control ==
  V : Inport
  Add : Sum  Inputs=-+
  Constant : Constant  Value=[P0 -Q0]
  Gain2 : Gain  Gain=1/tau_rms
  Integrator : Integrator  InitialCondition=1
  Product : Product  Inputs=/*
  Sqrt : Sqrt  SaturateOnIntegerOverflow=on
  Square : Math  Operator=square  SaturateOnIntegerOverflow=on
  Sum of Elements : Sum  Inputs=+
  i_dqref : Outport
  wires:
  Integrator/1 -> Product/1, Add/1
  Constant/1 -> Product/2
  Square/1 -> Sum of Elements/1
  Add/1 -> Gain2/1
  Sum of Elements/1 -> Sqrt/1
  Sqrt/1 -> Add/2
  Gain2/1 -> Integrator/1
  Product/1 -> i_dqref/1
  V/1 -> Square/1

== system device_library/device_SH_inverter/Inverse Park ==
  Vdq_cmd : Inport
  delta_PLL : Inport  Port=2
  Constant : Constant  Value=0
  Gain : Gain  Gain=base.V*sqrt(2/3)
  Mux : Mux  Inputs=2
  dq0 to abc : spsdq0toabcLib/dq0 to abc  Alignment=90 degrees behind phase A axis
  Vabc_cmd : Outport
  wires:
  Mux/1 -> dq0 to abc/1
  delta_PLL/1 -> dq0 to abc/2
  dq0 to abc/1 -> Gain/1
  Gain/1 -> Vabc_cmd/1
  Constant/1 -> Mux/2
  Vdq_cmd/1 -> Mux/1

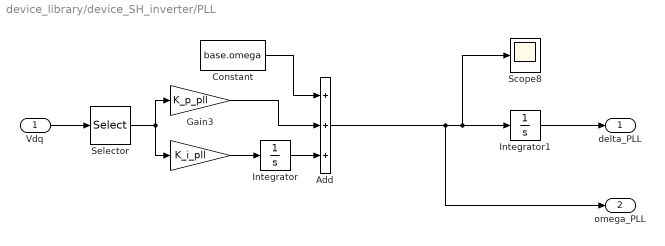
== system device_library/device_SH_inverter/PLL ==
  Vdq : Inport
  " " : Gain  Gain=K_i_pll
  Add : Sum  Inputs=+++
  Constant : Constant  Value=base.omega
  Gain3 : Gain  Gain=K_p_pll
  Integrator : Integrator
  Integrator1 : Integrator
  Scope8 : Scope
  Selector : Selector  InputPortWidth=2  IndexOptions=Index vector (dialog)  Indices=[2]  OutputSizes=1
  delta_PLL : Outport
  omega_PLL : Outport  Port=2
  wires:
  Add/1 -> omega_PLL/1, Integrator1/1, Scope8/1
  Integrator/1 -> Add/3
  Selector/1 -> Gain3/1, " "/1
  " "/1 -> Integrator/1
  Vdq/1 -> Selector/1
  Integrator1/1 -> delta_PLL/1
  Gain3/1 -> Add/2
  Constant/1 -> Add/1

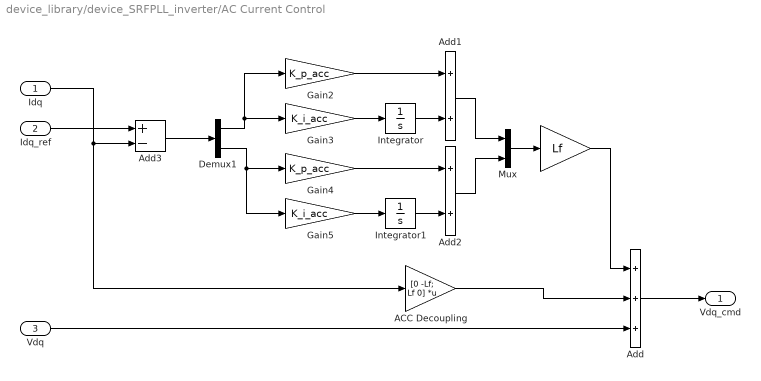
== system device_library/device_SRFPLL_inverter/AC Current Control ==
  Idq : Inport
  Idq_ref : Inport  Port=2
  Vdq : Inport  Port=3
  "  " : Gain  Gain=Lf
  ACC Decoupling : Gain  Gain=[0 -Lf; Lf 0]  Multiplication=Matrix(K*u) (u vector)
  Add : Sum  Inputs=3
  Add1 : Sum
  Add2 : Sum
  Add3 : Sum  Inputs=+-
  Demux1 : Demux  Outputs=2
  Gain2 : Gain  Gain=K_p_acc
  Gain3 : Gain  Gain=K_i_acc
  Gain4 : Gain  Gain=K_p_acc
  Gain5 : Gain  Gain=K_i_acc
  Integrator : Integrator
  Integrator1 : Integrator
  Mux : Mux  Inputs=2
  Vdq_cmd : Outport
  wires:
  "  "/1 -> Add/1
  Mux/1 -> "  "/1
  Demux1/2 -> Gain4/1, Gain5/1
  Add3/1 -> Demux1/1
  Gain4/1 -> Add2/1
  Add2/1 -> Mux/2
  Gain5/1 -> Integrator1/1
  Gain3/1 -> Integrator/1
  Add1/1 -> Mux/1
  Gain2/1 -> Add1/1
  Integrator/1 -> Add1/2
  Integrator1/1 -> Add2/2
  Demux1/1 -> Gain3/1, Gain2/1
  Add/1 -> Vdq_cmd/1
  Idq/1 -> ACC Decoupling/1, Add3/2
  Idq_ref/1 -> Add3/1
  ACC Decoupling/1 -> Add/2
  Vdq/1 -> Add/3

== system device_library/device_SRFPLL_inverter/Inverse Park ==
  Vdq_cmd : Inport
  delta_PLL : Inport  Port=2
  Constant : Constant  Value=0
  Gain : Gain  Gain=base.V*sqrt(2/3)
  Mux : Mux  Inputs=2
  dq0 to abc : spsdq0toabcLib/dq0 to abc  Alignment=90 degrees behind phase A axis
  Vabc_cmd : Outport
  wires:
  Mux/1 -> dq0 to abc/1
  delta_PLL/1 -> dq0 to abc/2
  dq0 to abc/1 -> Gain/1
  Gain/1 -> Vabc_cmd/1
  Constant/1 -> Mux/2
  Vdq_cmd/1 -> Mux/1

== system device_library/device_SRFPLL_inverter/PLL ==
  Vdq : Inport
  " " : Gain  Gain=K_i_pll
  Add : Sum  Inputs=+++
  Constant : Constant  Value=base.omega
  Gain3 : Gain  Gain=K_p_pll
  Integrator : Integrator
  Integrator1 : Integrator
  Scope8 : Scope
  Selector : Selector  InputPortWidth=2  IndexOptions=Index vector (dialog)  Indices=[2]  OutputSizes=1
  delta_PLL : Outport
  omega_PLL : Outport  Port=2
  wires:
  Add/1 -> omega_PLL/1, Integrator1/1, Scope8/1
  Integrator/1 -> Add/3
  Selector/1 -> Gain3/1, " "/1
  " "/1 -> Integrator/1
  Vdq/1 -> Selector/1
  Integrator1/1 -> delta_PLL/1
  Gain3/1 -> Add/2
  Constant/1 -> Add/1
